simulink model "cruiseControlModel2018b"  (R2022b)
settings: Solver=ode4  StartTime=0.0  StopTime=Tend  FixedStep=1  RelTol=1e-3
values from neighbouring files (symbols this model uses):
  roadGrade =     [roadGradeLookup.mat]
undefined symbols (not defined in the file or in its folder): a, Af, b, Cd, F_FF, g, gradeFlag, ki, Kp, M_tot, M_veh, rho, V0, V_FF, Vstep
settings Model: Creator=stockar.1  LastModifiedBy=77dal
settings SolverCC: AlgebraicLoopSolver=TrustRegion
settings DebuggingCC: UnconnectedInputMsg=warning  UnconnectedOutputMsg=warning  UnconnectedLineMsg=warning  SFMachineParentedDataDiag=warning  ArithmeticOperatorsInVariantConditions=warning
settings ModelReferenceCC: EnableRefExpFcnMdlSchedulingChecks=on
settings SFSimCC: CustomCodeUndefinedFunction=UseInterfaceOnly

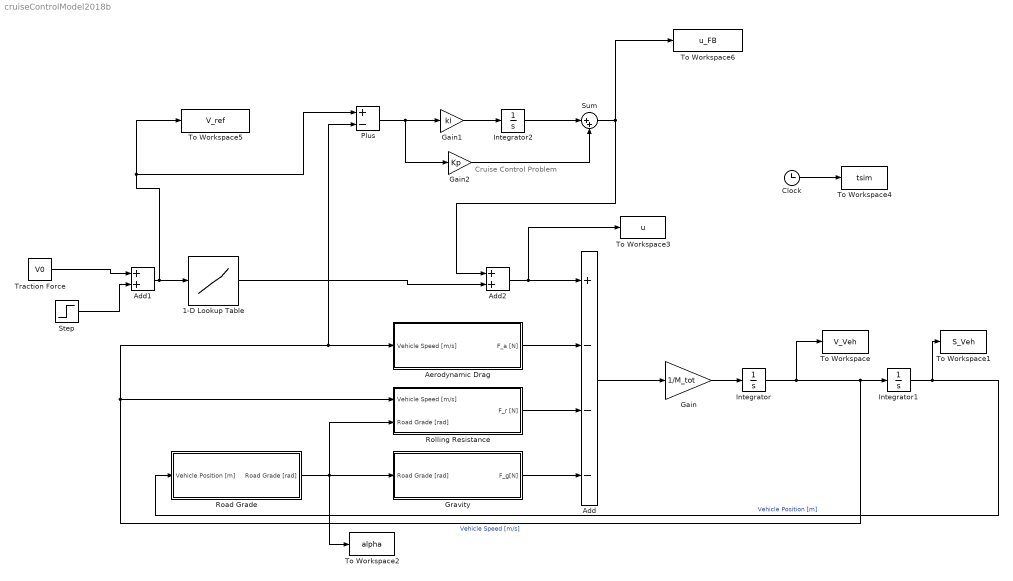
== system cruiseControlModel2018b ==
  note: Cruise Control Problem
  1-D Lookup Table : Lookup_n-D  NumberOfTableDimensions=1  BreakpointsForDimension1=V_FF  Table=F_FF  InternalRulePriority=Speed  RndMeth=Simplest
  Add : Sum  Inputs=+---
  Add1 : Sum
  Add2 : Sum
  Aerodynamic Drag : Subsystem
  Clock : Clock
  Gain : Gain  Gain=1/M_tot
  Gain1 : Gain  Gain=ki
  Gain2 : Gain  Gain=Kp
  Gravity : Subsystem
  Integrator : Integrator  InitialCondition=V0
  Integrator1 : Integrator
  Integrator2 : Integrator
  Plus : Sum  Inputs=+-
  Road Grade : Subsystem
  Rolling Resistance : Subsystem
  Step : Step  Time=200  After=Vstep  SampleTime=0
  Sum : Sum  Inputs=|++
  To Workspace : ToWorkspace  VariableName=V_Veh  SampleTime=-1
  To Workspace1 : ToWorkspace  VariableName=S_Veh  SampleTime=-1
  To Workspace2 : ToWorkspace  VariableName=alpha  SampleTime=-1
  To Workspace3 : ToWorkspace  VariableName=u  SampleTime=-1
  To Workspace4 : ToWorkspace  VariableName=tsim  SampleTime=-1
  To Workspace5 : ToWorkspace  VariableName=V_ref  SampleTime=-1
  To Workspace6 : ToWorkspace  VariableName=u_FB  SampleTime=-1
  Traction Force : Constant  Value=V0
  wires:
  Gain/1 -> Integrator/1
  Add/1 -> Gain/1
  Integrator/1 -> To Workspace/1, Rolling Resistance/1(Vehicle Speed [m/s]), Plus/2, Aerodynamic Drag/1(Vehicle Speed [m/s]), Integrator1/1  "Vehicle Speed [m/s]"
  Integrator1/1 -> To Workspace1/1, Road Grade/1(Vehicle Position [m])  "Vehicle Position [m]"
  Road Grade/1(Road Grade [rad]) -> To Workspace2/1, Rolling Resistance/2(Road Grade [rad]), Gravity/1(Road Grade [rad])
  Aerodynamic Drag/1(F_a [N]) -> Add/2
  Rolling Resistance/1(F_r [N]) -> Add/3
  Gravity/1(F_g[N]) -> Add/4
  Clock/1 -> To Workspace4/1
  Traction Force/1 -> Add1/1
  Step/1 -> Add1/2
  Add1/1 -> 1-D Lookup Table/1, To Workspace5/1, Plus/1
  Gain1/1 -> Integrator2/1
  Integrator2/1 -> Sum/1
  Gain2/1 -> Sum/2
  Plus/1 -> Gain2/1, Gain1/1
  Sum/1 -> Add2/1, To Workspace6/1
  1-D Lookup Table/1 -> Add2/2
  Add2/1 -> To Workspace3/1, Add/1

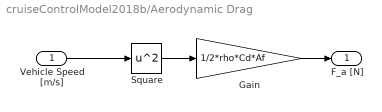
== system cruiseControlModel2018b/Aerodynamic Drag ==
  Vehicle Speed [m/s] : Inport
  Gain : Gain  Gain=1/2*rho*Cd*Af
  Square : Math  Operator=square  SignedPower=on
  F_a [N] : Outport
  wires:
  Vehicle Speed [m/s]/1 -> Square/1
  Square/1 -> Gain/1
  Gain/1 -> F_a [N]/1

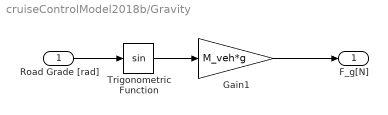
== system cruiseControlModel2018b/Gravity ==
  Road Grade [rad] : Inport
  Gain1 : Gain  Gain=M_veh*g
  Trigonometric Function : Trigonometry
  F_g[N] : Outport
  wires:
  Gain1/1 -> F_g[N]/1
  Road Grade [rad]/1 -> Trigonometric Function/1
  Trigonometric Function/1 -> Gain1/1

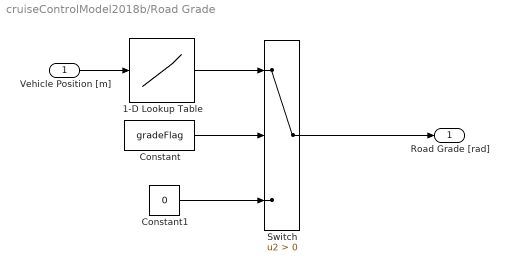
== system cruiseControlModel2018b/Road Grade ==
  Vehicle Position [m] : Inport
  1-D Lookup Table : Lookup_n-D  NumberOfTableDimensions=1  BreakpointsForDimension1=roadGrade.position  Table=roadGrade.alpha  InternalRulePriority=Speed  RndMeth=Simplest
  Constant : Constant  Value=gradeFlag
  Constant1 : Constant  Value=0
  Switch : Switch  Criteria=u2 > Threshold  SaturateOnIntegerOverflow=off  InputSameDT=off
  Road Grade [rad] : Outport
  wires:
  Vehicle Position [m]/1 -> 1-D Lookup Table/1
  1-D Lookup Table/1 -> Switch/1
  Constant/1 -> Switch/2
  Constant1/1 -> Switch/3
  Switch/1 -> Road Grade [rad]/1

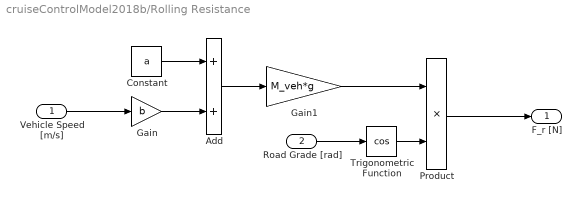
== system cruiseControlModel2018b/Rolling Resistance ==
  Vehicle Speed [m/s] : Inport
  Road Grade [rad] : Inport  Port=2
  Add : Sum
  Constant : Constant  Value=a
  Gain : Gain  Gain=b
  Gain1 : Gain  Gain=M_veh*g
  Product : Product
  Trigonometric Function : Trigonometry  Operator=cos
  F_r [N] : Outport
  wires:
  Product/1 -> F_r [N]/1
  Vehicle Speed [m/s]/1 -> Gain/1
  Gain/1 -> Add/2
  Constant/1 -> Add/1
  Add/1 -> Gain1/1
  Gain1/1 -> Product/1
  Road Grade [rad]/1 -> Trigonometric Function/1
  Trigonometric Function/1 -> Product/2
